simulink model "test_model_2"  (R2019a)
settings: Solver=VariableStepAuto  StartTime=0.0  StopTime=100  RelTol=1e-3
settings Model: Creator=Yusuf  LastModifiedBy=Yusuf

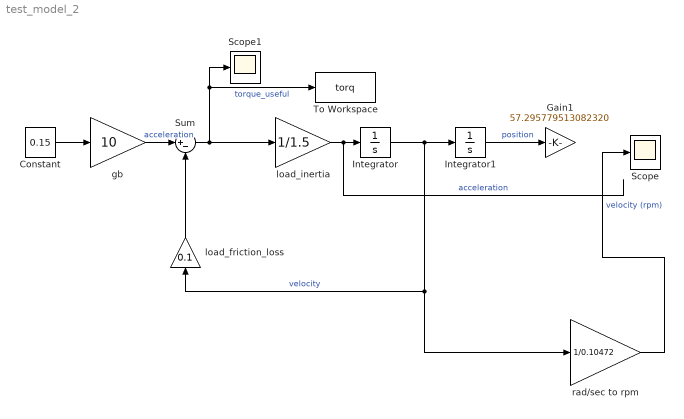
== system test_model_2 ==
  Constant : Constant  Value=0.15
  Gain1 : Gain  Gain=57.295779513082320
  Integrator : Integrator
  Integrator1 : Integrator
  Scope : Scope  NumInputPorts=3
  Scope1 : Scope
  Sum : Sum  Inputs=|+-
  To Workspace : ToWorkspace  VariableName=torq  SaveFormat=Timeseries  SampleTime=-1
  gb : Gain  Gain=10
  load_friction_loss : Gain  Gain=0.1
  load_inertia : Gain  Gain=1/1.5
  rad/sec to rpm : Gain  Gain=1/0.10472
  wires:
  Sum/1 -> To Workspace/1, Scope1/1, load_inertia/1  "torque_useful"
  load_inertia/1 -> Integrator/1  "acceleration"
  Integrator/1 -> load_friction_loss/1, rad/sec to rpm/1, Integrator1/1  "velocity"
  Constant/1 -> gb/1
  rad/sec to rpm/1 -> Scope/2  "velocity (rpm)"
  Integrator1/1 -> Gain1/1  "position"
  load_friction_loss/1 -> Sum/2
  gb/1 -> Sum/1  "acceleration"
